simulink model "DKTN_CKI"  (R2023a)
settings: Solver=VariableStepAuto  StartTime=0.0  StopTime=100  FixedStep=0.005  RelTol=1e-3
libraries: SignalEditorBlockLib x2, simulink x1, cstblocks x1, slpidlib x1
settings Model: Creator=FPTSHOP  LastModifiedBy=FPTSHOP

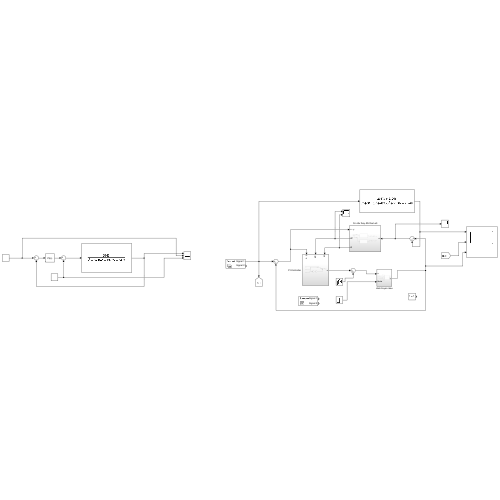
[thumbnail: Simulink's stored preview of the top-level diagram]
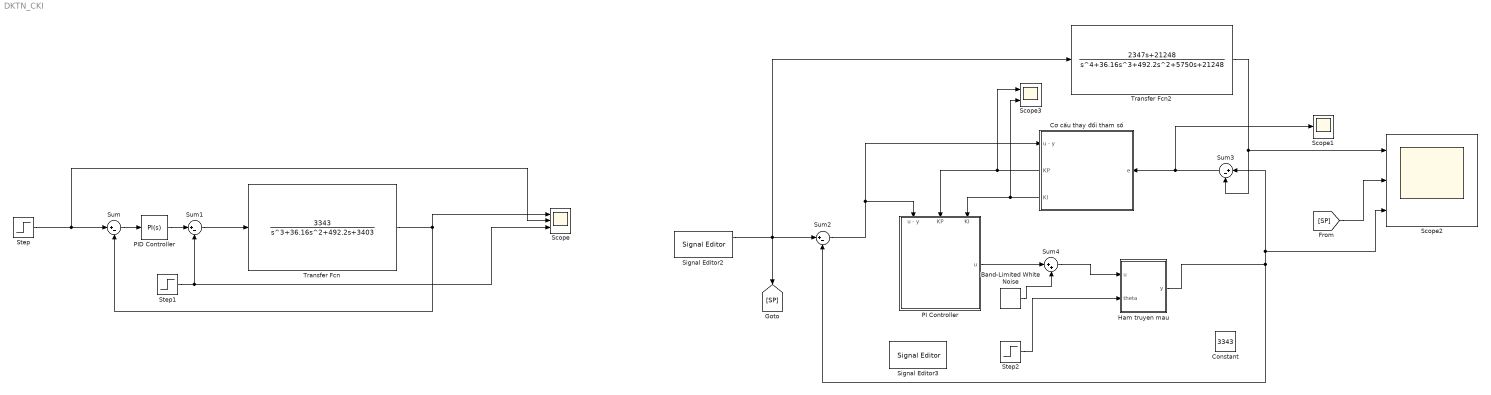
== system DKTN_CKI ==
  Band-Limited White Noise : simulink/Sources/Band-Limited White Noise  Cov=[0.0001]  Ts=0.1  seed=[23341]
  Constant : Constant  Value=3343
  Cơ cấu thay đổi tham số : Subsystem
      settings: PortSchema="{\"entries\":[{\"content\":{\"sides\":[{\"content\":{\"connectorIds\":[\"In1\"]},\"type\":\"ConnectorPlacement.EquallySpacedRectSide\",\"uuid\":\"80899429-ec5e-4ea6-9130-530fe1f37aef\"},{\"content\":{\"connectorIds\":[\"In2\",\"Out1\",\"Out2\"],\"side\":\"RIGHT\"},\"type\":\"ConnectorPlacement.EquallySpacedRectSide\",\"uuid\":\"4a2de49c-21b3-4ae3-b9e0-d77aef8f9de0\"},{\"content\":{\"side\":\"TOP\"},\"type\":\"ConnectorPlacement.EquallySpacedRectSide\",\"uuid\":\"a7b60cec-568b-41d4-926d-6ff42a0e1872\"},{\"content\":{\"side\":\"BOTTOM\"},\"type\":\"ConnectorPlacement.EquallySpacedRectSide\",\"uuid\":\"44227394-6553-42ce-9b91-3aff6074a502\"}]},\"type\":\"ConnectorPlacement.EquallySpacedConnector\",\"uuid\":\"655fcbc3-75b2-4ba4-9e50-e4789fbe396c\"}],\"packageUris\":[\"http://schema.mathworks.com/mf0/Connector/R2020b\"],\"version\":\"1.0\"}"
  Ham truyen mau : Subsystem
  PI Controller : Subsystem
      settings: PortSchema="{\"entries\":[{\"content\":{\"sides\":[{\"content\":{\"connectorIds\":[\"In1\",\"In2\",\"In3\"]},\"type\":\"ConnectorPlacement.EquallySpacedRectSide\",\"uuid\":\"dddaaed2-e507-451a-921f-c04901101d86\"},{\"content\":{\"side\":\"RIGHT\"},\"type\":\"ConnectorPlacement.EquallySpacedRectSide\",\"uuid\":\"ae8720e4-d060-4dea-b1b4-5825fbf776f2\"},{\"content\":{\"side\":\"TOP\"},\"type\":\"ConnectorPlacement.EquallySpacedRectSide\",\"uuid\":\"05c90be4-7f2e-46e3-b0ab-720f61a4a343\"},{\"content\":{\"connectorIds\":[\"Out1\"],\"side\":\"BOTTOM\"},\"type\":\"ConnectorPlacement.EquallySpacedRectSide\",\"uuid\":\"f7a2217c-f25e-4afe-a869-2b8c8d87a3a7\"}]},\"type\":\"ConnectorPlacement.EquallySpacedConnector\",\"uuid\":\"e4383ad1-63b6-41a4-973a-f7aa36cab285\"}],\"packageUris\":[\"http://schema.mathworks.com/mf0/Connector/R2020b\"],\"version\":\"1.0\"}"
  PID Controller : slpidlib/PID Controller  Controller=PI  Form=Parallel  TimeDomain=Continuous-time  UseExternalTs=off  SampleTime=-1  IntegratorMethod=Forward Euler  FilterMethod=Forward Euler  ControllerParametersSource=internal  P=0.70230248213526  I=6.35759576592185  UseKiTs=off  D=0  N=100  UseFilter=on  TunerSelectOption=Transfer Function Based (PID Tuner App)  InitialConditionSource=internal  InitialConditionForIntegrator=0  InitialConditionForFilter=0  DifferentiatorICPrevScaledInput=0  ExternalReset=none  TrackingMode=off  Kt=1  LimitOutput=off  SatLimitsSource=internal  UpperSaturationLimit=inf  LowerSaturationLimit=-inf  LinearizeAsGain=on  AntiWindupMode=none  Kb=1  LimitIntegrator=off  UpperIntegratorSaturationLimit=inf  LowerIntegratorSaturationLimit=-inf  POutMin=[]  POutMax=[]  IOutMin=[]  IOutMax=[]  DOutMin=[]  DOutMax=[]  NOutMin=[]  NOutMax=[]  SumOutMin=[]  SumOutMax=[]  SaturationOutMin=[]  SaturationOutMax=[]  PParamMin=[]  PParamMax=[]  IParamMin=[]  IParamMax=[]  DParamMin=[]  DParamMax=[]  NParamMin=[]  NParamMax=[]  KbParamMin=[]  KbParamMax=[]  KtParamMin=[]  KtParamMax=[]  KbOutMin=[]  KbOutMax=[]  KtOutMin=[]  KtOutMax=[]  IntegratorOutMin=[]  IntegratorOutMax=[]  FilterOutMin=[]  FilterOutMax=[]  SumI1OutMin=[]  SumI1OutMax=[]  SumI2OutMin=[]  SumI2OutMax=[]  SumI3OutMin=[]  SumI3OutMax=[]  SumI4OutMin=[]  SumI4OutMax=[]  SumDOutMin=[]  SumDOutMax=[]  DifferentiatorOutMin=[]  DifferentiatorOutMax=[]  FilterDiffOutCoefMin=[]  FilterDiffOutCoefMax=[]  ReciprocalOutMin=[]  ReciprocalOutMax=[]  SumDenOutMin=[]  SumDenOutMax=[]  SumNumOutMin=[]  SumNumOutMax=[]  DivideOutMin=[]  DivideOutMax=[]  UdiffTsProdOutMin=[]  UdiffTsProdOutMax=[]  NTsProdOutMin=[]  NTsProdOutMax=[]  UintegralTsProdOutMin=[]  UintegralTsProdOutMax=[]  UngainTsProdOutMin=[]  UngainTsProdOutMax=[]  ClampingZeroOutDataTypeStr=Inherit: Inherit via back propagation  ClampingZeroOutMin=[]  ClampingZeroOutMax=[]  FilterDenConstantOutDataTypeStr=Inherit: Inherit via back propagation  FilterDenConstantOutMin=[]  FilterDenConstantOutMax=[]  PCopyOutDataTypeStr=Inherit: Inherit via back propagation  PCopyOutMin=[]  PCopyOutMax=[]  NCopyOutDataTypeStr=Inherit: Inherit via back propagation  NCopyOutMin=[]  NCopyOutMax=[]  IntegratorContinuousStateAttributes=''  IntegratorStateMustResolveToSignalObject=off  IntegratorRTWStateStorageClass=Auto  FilterContinuousStateAttributes=''  FilterStateMustResolveToSignalObject=off  FilterRTWStateStorageClass=Auto  ParallelPVariant=InternalParameters  IdealPVariant=Disabled  IVariant=InternalParameters  DVariant=Disabled  IntegratorVariant=Continuous  SatVariant=Disabled  AWVariant=Passthrough  PCopyVariant=Disabled  TRVariant=Disabled  FdbkBlocksVariant=Forward  IdealPFdbkVariant=Disabled  SatFdbkVariant=Disabled  DerivativeFilterVariant=Disabled  NVariant=Disabled  NCopyVariant=Disabled_SignalSpec  FilterICVariant=Disabled  IntegratorICVariant=InternalICs  ExternalResetVariant=Disabled  TRSumVariant=Passthrough  SumFdbkVariant=Disabled  SumVariant=Sum_PI  TsampFilterVariant=InternalTs  TsampNgainVariant=Passthrough  TsampIntegralVariant=Disabled_SignalSpec  ExternalSaturationOutDataTypeStr=Inherit: Same as second input
  Scope : Scope  NumInputPorts=3
  Scope1 : Scope
  Scope2 : Scope  NumInputPorts=3
  Scope3 : Scope  NumInputPorts=2
  Signal Editor2 : SignalEditorBlockLib/Signal Editor  FileName=I:\DUT\DK Thich Nghi\CUOIKI\signal.mat  ActiveScenario=Scenario  ActiveSignal=Signal 1  IsBus=off  OutputBusObjectStr=Bus: BusObject  SampleTime=0  Interpolate=off  ZeroCross=off  OutputAfterFinalValue=Setting to zero  Unit=inherit  PreserveSignalName=on  ApplySigPropsToAllScenarios=on
  Signal Editor3 : SignalEditorBlockLib/Signal Editor  FileName=I:\DUT\DK Thich Nghi\CUOIKI\signal.mat  ActiveScenario=Scenario  ActiveSignal=Signal 1  IsBus=off  OutputBusObjectStr=Bus: BusObject  SampleTime=0  Interpolate=off  ZeroCross=off  OutputAfterFinalValue=Setting to zero  Unit=inherit  PreserveSignalName=on  ApplySigPropsToAllScenarios=on
  Step : Step  Time=10  SampleTime=0
  Step1 : Step  Time=20  After=2  SampleTime=0
  Step2 : Step  Time=40  Before=3343  After=4000  SampleTime=0
  Sum{,1..3} (4 alike) : Sum  Inputs=|+-
  Sum4 : Sum  Inputs=|++
  Transfer Fcn : TransferFcn  Numerator=[3343]  Denominator=[1 36.16 492.2 3403]
  Transfer Fcn2 : TransferFcn  Numerator=[2347 21248]  Denominator=[1 36.16 492.2 5750 21248]
  wires:
  Step/1 -> Sum/1, Scope/2
  Sum/1 -> PID Controller/1
  Transfer Fcn/1 -> Sum/2, Scope/1
  PID Controller/1 -> Sum1/1
  Sum1/1 -> Transfer Fcn/1
  Step1/1 -> Scope/3, Sum1/2
  Sum3/1 -> Scope1/1, Cơ cấu thay đổi tham số/1(e)
  [SP] -> Scope2/2
  Ham truyen mau/1(y) -> Scope2/3, Sum3/1, Sum2/2
  Transfer Fcn2/1 -> Sum3/2, Scope2/1
  Cơ cấu thay đổi tham số/1(KP) -> Scope3/1, PI Controller/2(KP)
  Signal Editor2/1 -> [SP], Transfer Fcn2/1, Sum2/1
  Cơ cấu thay đổi tham số/2(KI) -> Scope3/2, PI Controller/3(KI)
  Sum2/1 -> PI Controller/1(u - y), Cơ cấu thay đổi tham số/2(u - y)
  Step2/1 -> Ham truyen mau/2(theta)
  PI Controller/1(u) -> Sum4/1
  Sum4/1 -> Ham truyen mau/1(u)
  Band-Limited White Noise/1 -> Sum4/2

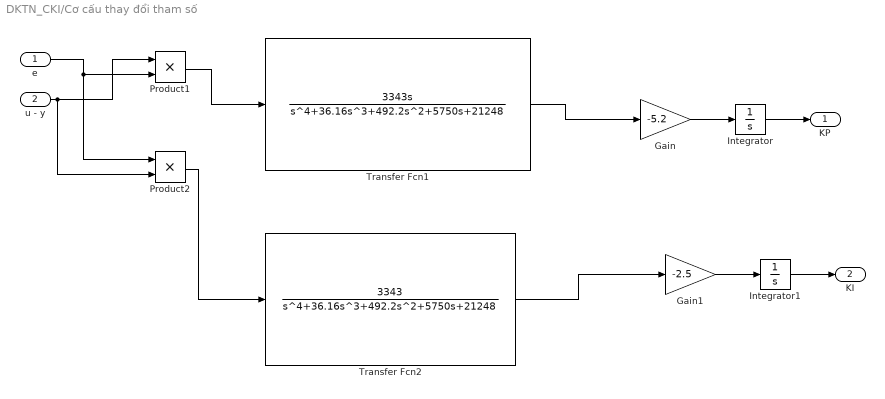
== system DKTN_CKI/Cơ cấu thay đổi tham số ==
  e : Inport
  u - y : Inport  Port=2
  Gain : Gain  Gain=-5.2
  Gain1 : Gain  Gain=-2.5
  Integrator : Integrator  InitialCondition=1.02
  Integrator1 : Integrator  InitialCondition=0.98
  Product1 : Product
  Product2 : Product
  Transfer Fcn1 : TransferFcn  Numerator=[3343 0]  Denominator=[1 36.16 492.2 5750 21248]
  Transfer Fcn2 : TransferFcn  Numerator=[3343]  Denominator=[1 36.16 492.2 5750 21248]
  KP : Outport
  KI : Outport  Port=2
  wires:
  Transfer Fcn1/1 -> Gain/1
  Gain/1 -> Integrator/1
  Integrator/1 -> KP/1
  Transfer Fcn2/1 -> Gain1/1
  Gain1/1 -> Integrator1/1
  Integrator1/1 -> KI/1
  e/1 -> Product2/1, Product1/2
  u - y/1 -> Product2/2, Product1/1
  Product1/1 -> Transfer Fcn1/1
  Product2/1 -> Transfer Fcn2/1

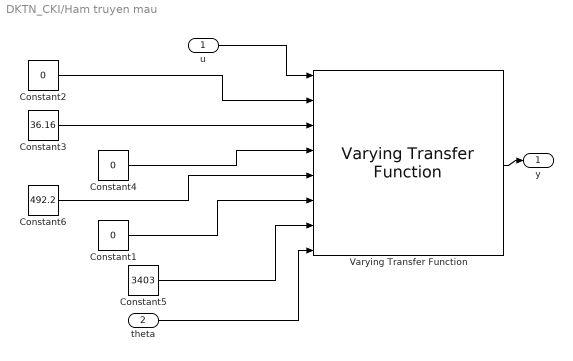
== system DKTN_CKI/Ham truyen mau ==
  u : Inport
  theta : Inport  Port=2
  Constant1 : Constant  Value=0
  Constant2 : Constant  Value=0
  Constant3 : Constant  Value=36.16
  Constant4 : Constant  Value=0
  Constant5 : Constant  Value=3403
  Constant6 : Constant  Value=492.2
  Varying Transfer Function : cstblocks/Linear Parameter Varying/Varying Transfer Function  N=3  Feedthrough=on
  y : Outport
  wires:
  Varying Transfer Function/1 -> y/1
  u/1 -> Varying Transfer Function/1
  Constant2/1 -> Varying Transfer Function/2
  Constant1/1 -> Varying Transfer Function/6
  theta/1 -> Varying Transfer Function/8
  Constant3/1 -> Varying Transfer Function/3
  Constant4/1 -> Varying Transfer Function/4
  Constant5/1 -> Varying Transfer Function/7
  Constant6/1 -> Varying Transfer Function/5

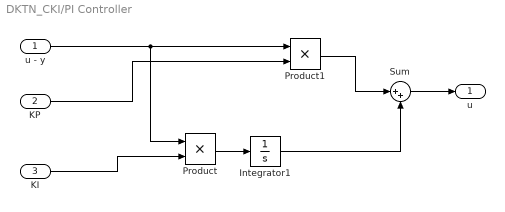
== system DKTN_CKI/PI Controller ==
  u - y : Inport
  KP : Inport  Port=2
  KI : Inport  Port=3
  Integrator1 : Integrator
  Product : Product
  Product1 : Product
  Sum : Sum  Inputs=|++
  u : Outport
  wires:
  KP/1 -> Product1/2
  u - y/1 -> Product/1, Product1/1
  Sum/1 -> u/1
  Product1/1 -> Sum/1
  KI/1 -> Product/2
  Product/1 -> Integrator1/1
  Integrator1/1 -> Sum/2
